simulink model "Minimos_Cuadrados_directo"  (R2018a)
settings: Solver=VariableStepAuto  StartTime=0.0  StopTime=10.0  RelTol=1e-3
values from neighbouring files (symbols this model uses):
  b = 0.05    [Ppendulo.m]
  g = 9.81    [Ppendulo.m]
  l = 0.45    [Ppendulo.m]
  m = 0.5    [Ppendulo.m]
  M = 2    [Ppendulo.m]
libraries: dspinverses x1
settings Model: Creator=Omie-PC  LastModifiedBy=Benjamin Nicolas

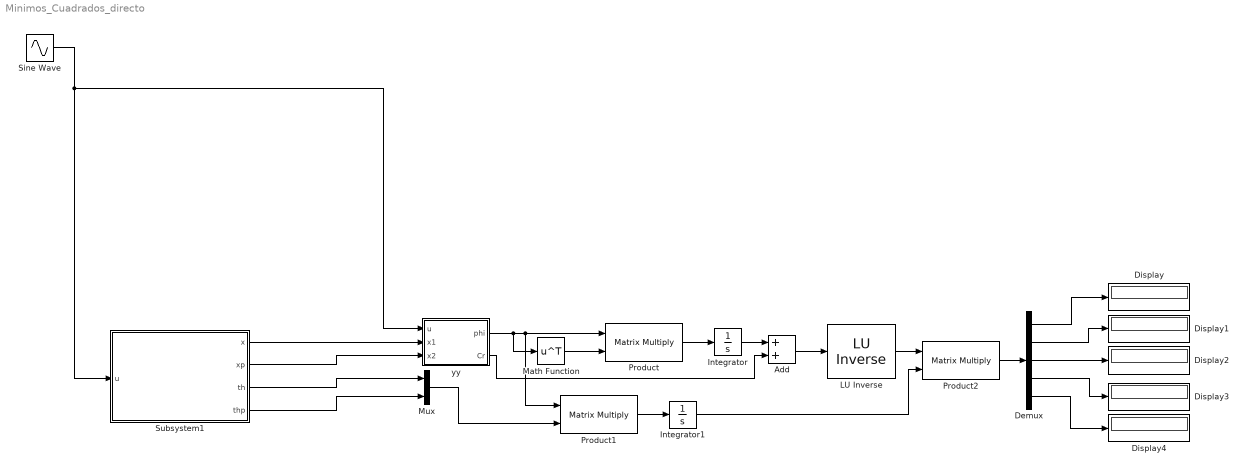
== system Minimos_Cuadrados_directo ==
  " LU Inverse" : dspinverses/ LU Inverse
      settings: SourceProductName=DSP System Toolbox
  Add : Sum
  Demux : Demux  Outputs=5
  Display{,1..4} (5 alike) : Display
  Integrator : Integrator
  Integrator1 : Integrator
  Math Function : Math  Operator=transpose  SaturateOnIntegerOverflow=on
  Mux : Mux  Inputs=2
  Product : Product  Multiplication=Matrix(*)
  Product1 : Product  Multiplication=Matrix(*)
  Product2 : Product  Multiplication=Matrix(*)
  Sine Wave : Sin  Frequency=1000  SampleTime=0
  Subsystem1 : Subsystem
  yy : MATLAB Function  TreatAsAtomicUnit=on
  wires:
  yy/1(phi) -> Math Function/1, Product/1, Product1/1
  Math Function/1 -> Product/2
  Subsystem1/1(x) -> yy/2(x1)
  Subsystem1/2(xp) -> yy/3(x2)
  Product/1 -> Integrator/1
  Sine Wave/1 -> Subsystem1/1(u), yy/1(u)
  Subsystem1/3(th) -> Mux/1
  Subsystem1/4(thp) -> Mux/2
  Mux/1 -> Product1/2
  Product1/1 -> Integrator1/1
  Integrator/1 -> Add/1
  Add/1 -> " LU Inverse"/1
  " LU Inverse"/1 -> Product2/1
  Integrator1/1 -> Product2/2
  Product2/1 -> Demux/1
  Demux/5 -> Display4/1
  Demux/4 -> Display3/1
  Demux/3 -> Display2/1
  Demux/2 -> Display1/1
  Demux/1 -> Display/1
  yy/2(Cr) -> Add/2

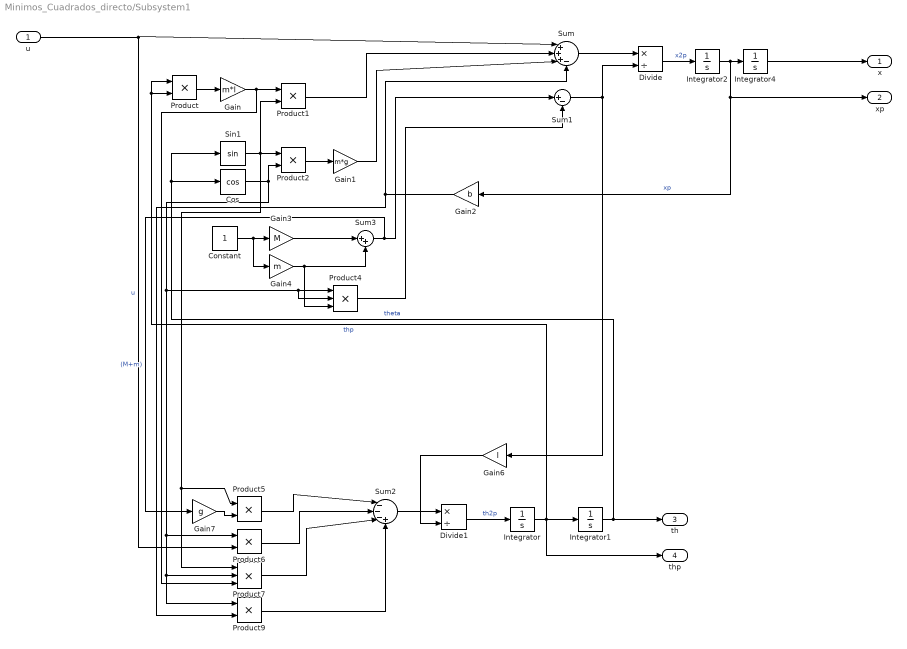
== system Minimos_Cuadrados_directo/Subsystem1 ==
  u : Inport
  Constant : Constant
  Cos : Trigonometry  Operator=cos
  Divide : Product  Inputs=*/
  Divide1 : Product  Inputs=*/
  Gain : Gain  Gain=m*l
  Gain1 : Gain  Gain=m*g
  Gain2 : Gain  Gain=b
  Gain3 : Gain  Gain=M
  Gain4 : Gain  Gain=m
  Gain6 : Gain  Gain=l
  Gain7 : Gain  Gain=g
  Integrator : Integrator
  Integrator1 : Integrator  InitialCondition=pi
  Integrator2 : Integrator
  Integrator4 : Integrator
  Product{,1..2,5..6,9} (6 alike) : Product
  Product4 : Product  Inputs=3
  Product7 : Product  Inputs=3
  Sin1 : Trigonometry
  Sum : Sum  Inputs=|+++-
  Sum1 : Sum  Inputs=|+-
  Sum2 : Sum  Inputs=|---+
  Sum3 : Sum  Inputs=|++
  x : Outport
  xp : Outport  Port=2
  th : Outport  Port=3
  thp : Outport  Port=4
  wires:
  u/1 -> Sum/1, Product6/2  "u"
  Product2/1 -> Gain1/1
  Gain1/1 -> Sum/3
  Constant/1 -> Gain4/1, Gain3/1
  Sin1/1 -> Product1/2, Product7/1, Product5/1, Product2/1
  Integrator1/1 -> Sin1/1, Cos/1, th/1  "theta"
  Integrator2/1 -> Gain2/1, xp/1, Integrator4/1  "xp"
  Divide1/1 -> Integrator/1  "th2p"
  Integrator/1 -> Product/2, Product/1, thp/1, Integrator1/1  "thp"
  Product1/1 -> Sum/2
  Gain7/1 -> Product5/2
  Cos/1 -> Product9/1, Product7/2, Product6/1, Product4/2, Product4/1, Product2/2
  Sum1/1 -> Gain6/1, Divide/2
  Gain3/1 -> Sum3/1
  Divide/1 -> Integrator2/1  "x2p"
  Sum3/1 -> Gain7/1, Sum1/1  "(M+m)"
  Gain6/1 -> Divide1/2
  Product9/1 -> Sum2/4
  Gain2/1 -> Product9/2, Sum/4
  Product5/1 -> Sum2/1
  Sum2/1 -> Divide1/1
  Gain4/1 -> Product4/3, Sum3/2
  Product6/1 -> Sum2/2
  Integrator4/1 -> x/1
  Product4/1 -> Sum1/2
  Sum/1 -> Divide/1
  Product7/1 -> Sum2/3
  Gain/1 -> Product7/3, Product1/1
  Product/1 -> Gain/1

== matlab function Minimos_Cuadrados_directo/yy ==
  data: u input; x1 input; phi output; x2 input; Cr output
function [phi,Cr]  = fcn(u,x1,x2)
k=0.1;
Cr=k*eye(5);
phi = [0,sin(x1);0,x2;0,tanh(x2);0,u;x2,0];
